simulink model "with_reference_input"  (R2014a)
settings: Solver=ode3  SolverMode=SingleTasking  StartTime=0.0  StopTime=20  RelTol=1e-3
values from neighbouring files (symbols this model uses):
  A_full = [Xu Xw 0 -g 0 ... (first row only)    [LQR_controller.m]
  B_full = [Xde;Zde;Mde;0;0]    [LQR_controller.m]
  K_full = lqr(A_full,B_full,[0 0 0 0 0;0 0 0 0 0;0 0 0 0 0;0 0 0 0 0;0 0 0 0 0.5],50)    [LQR_controller.m]
settings Model: ExtModeTrigDuration=2  Creator=Abdelrahman  LastModifiedBy=Abdelrahman
settings OptimizationCC: OptimizeModelRefInitCode=on  LifeSpan=1
settings DebuggingCC: UnderspecifiedInitializationDetection=Classic  SolverPrmCheckMsg=none
settings HardwareCC: ProdBitPerInt=16  ProdBitPerPointer=8  ProdIntDivRoundTo=Zero  ProdEndianess=LittleEndian  ProdWordSize=8  ProdHWDeviceType=Atmel->AVR
settings RTWCC: SystemTargetFile=realtime.tlc  GenerateMakefile=off  TemplateMakefile=realtime.tmf  Description=Run on Target Hardware  RTWVerbose=off  ProcessScript=realtime_make_rtw_hook
settings STFCustomTargetCC: TargetLibSuffix=.a  GenerateSampleERTMain=on  ConcurrentExecutionCompliant=off  GeneratePreprocessorConditionals=Use local settings  ERTCustomFileBanners=on  SupportNonInlinedSFcns=off  SupportVariableSizeSignals=on  MATLABClassNameForMDSCustomization=Simulink.SoftwareTarget.ERTCustomization  GRTInterface=off  SystemTargetFile=realtime.tlc
settings ERTTargetCC: CombineOutputUpdateFcns=off  SupportContinuousTime=on  SupportVariableSizeSignals=on  ExtModeTransport=3  ExtModeMexFile=ext_serial_win32_comm  ExtModeMexArgs=0 1 9600  ERTSrcFileBannerTemplate=realtime_code_template.cgt  ERTHdrFileBannerTemplate=realtime_code_template.cgt  ERTDataSrcFileTemplate=realtime_code_template.cgt  ERTDataHdrFileTemplate=realtime_code_template.cgt  ERTCustomFileTemplate=realtime_file_process.tlc

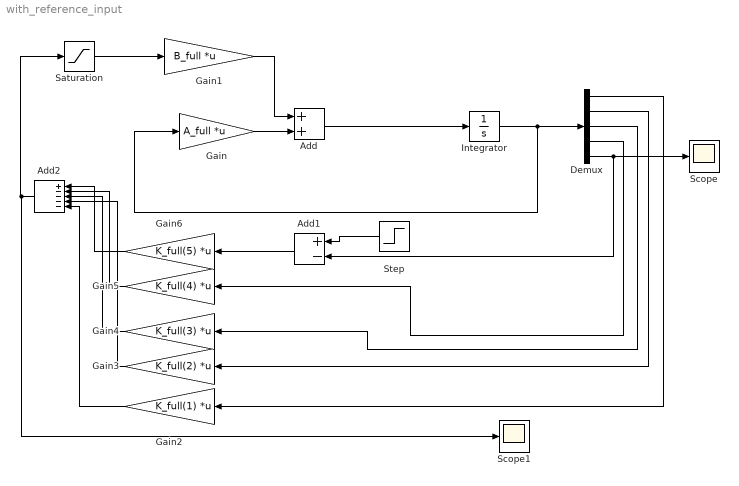
== system with_reference_input ==
  Add : Sum
  Add1 : Sum  Inputs=+-
  Add2 : Sum  Inputs=+----
  Demux : Demux  Outputs=5
  Gain : Gain  Gain=A_full  Multiplication=Matrix(K*u)
  Gain1 : Gain  Gain=B_full  Multiplication=Matrix(K*u)
  Gain2 : Gain  Gain=K_full(1)  Multiplication=Matrix(K*u)
  Gain3 : Gain  Gain=K_full(2)  Multiplication=Matrix(K*u)
  Gain4 : Gain  Gain=K_full(3)  Multiplication=Matrix(K*u)
  Gain5 : Gain  Gain=K_full(4)  Multiplication=Matrix(K*u)
  Gain6 : Gain  Gain=K_full(5)  Multiplication=Matrix(K*u)
  Integrator : Integrator  InitialCondition=1
  Saturation : Saturate
  Scope : Scope
      settings: TimeRange=10  YMin=0.9999999998750002  YMax=1.000000000125
  Scope1 : Scope
      settings: TimeRange=10  YMin=0.9999999998750002  YMax=1.000000000125
  Step : Step  After=100  SampleTime=0
  wires:
  Integrator/1 -> Demux/1, Gain/1
  Gain/1 -> Add/2
  Gain1/1 -> Add/1
  Add/1 -> Integrator/1
  Demux/1 -> Gain2/1
  Demux/2 -> Gain3/1
  Demux/3 -> Gain4/1
  Demux/4 -> Gain5/1
  Demux/5 -> Add1/2, Scope/1
  Step/1 -> Add1/1
  Gain6/1 -> Add2/1
  Gain5/1 -> Add2/2
  Gain4/1 -> Add2/3
  Gain3/1 -> Add2/4
  Gain2/1 -> Add2/5
  Add1/1 -> Gain6/1
  Add2/1 -> Scope1/1, Saturation/1
  Saturation/1 -> Gain1/1
